simulink model "realtime_PID"  (R2024b)
settings: Solver=ode5  StartTime=0.0  StopTime=10  FixedStep=0.001  RelTol=1e-3
values from neighbouring files (symbols this model uses):
  Beq = 1.223604206496999e-06    (= 1.2236042065e-06)    [DesignPart567.m]    (also in DesignPart9Sine.m; DesignPart9Step.m; Init.m; Real_time_parameter_estimation.m = (data.Beq_hat_pos + data.Beq_hat_neg)/2)
  k_drv = (1 + drv.R3/drv.R4) * drv.R2/(drv.R1 + drv.R2)    [Init.m]
  Kd = Kp * Td    [Init.m]
  Ki = Kp / Ti    [Init.m]
  Kp = deltak * cos(deltaphi)    [Init.m]
  Kw = 1/Tw    (= 33.3333333333)    [Init.m]
  rpm2rads = 2*pi/60    (= 0.10471975512)    [Init.m]
  Tau_sf = 0.005709536387019    (= 0.00570953638702)    [DesignPart567.m]    (also in DesignPart9Sine.m; DesignPart9Step.m; Init.m; State_space_1324.m)
  tl = 1/(3*wgc)    [Init.m]
undefined symbols (not defined in the file or in its folder): gbox, mot, National_Instruments, PCI, sens
libraries: sldrtlib x7, simulink x1
settings Model: SimulationMode=external  ExtModeTrigDuration=1000001  Creator=galeazzolu  LastModifiedBy=lucag
settings DataIOCC: ReturnWorkspaceOutputs=off
settings HardwareCC: ProdBitPerLong=64  ProdHWDeviceType=Intel->x86-64 (Linux 64)
settings RTWCC: Description=Simulink Desktop Real-Time  SystemTargetFile=sldrt.tlc  TemplateMakefile=sldrt.tmf  RTWCompilerOptimization=on
settings CodeAppCC: MaxIdLength=95
settings SimulinkDesktopRealTimeCC: TargetLibSuffix=_sldrt.a  TargetPreCompLibLocation=C:\Program Files\MATLAB\R2024b\toolbox\sldrt\lib\win64  ParMdlRefBuildCompliant=on

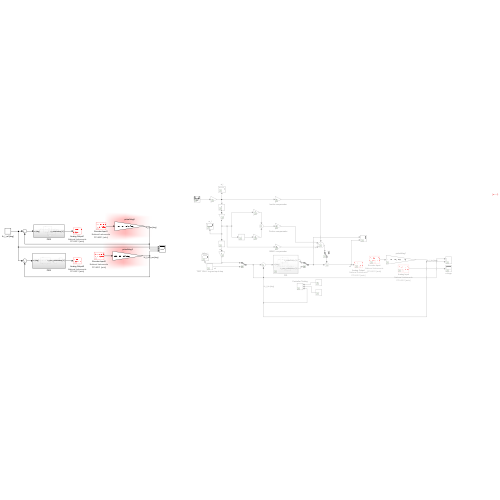
[thumbnail: Simulink's stored preview of the top-level diagram]
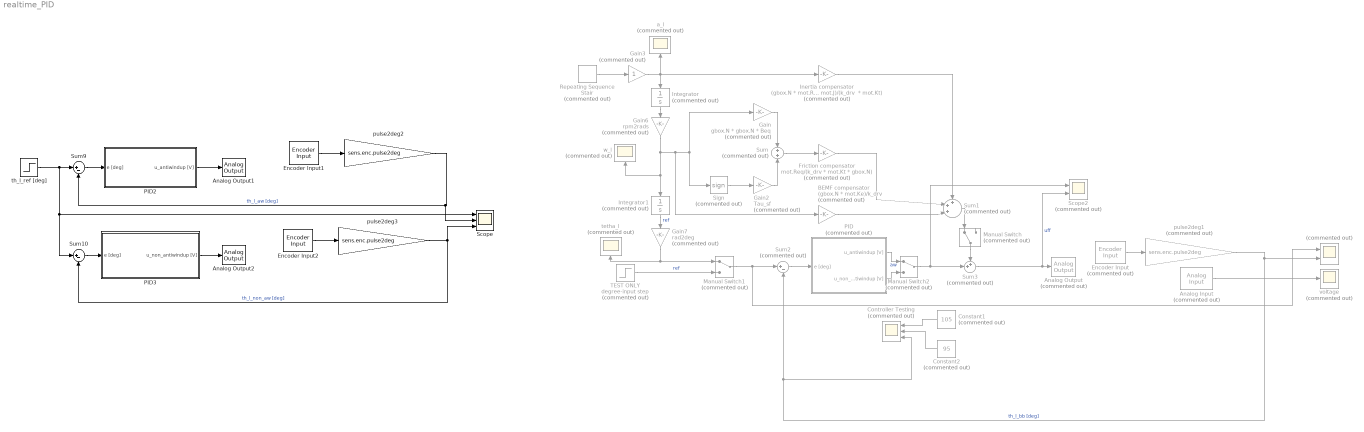
== system realtime_PID ==
  " " : Scope  Commented=on  NumInputPorts=2
  " a_l" : Scope  Commented=on
  " tetha_l" : Scope  Commented=on
  " w_l" : Scope  Commented=on
  Analog Input : sldrtlib/Analog Input  Commented=on  SampleTime=-1  MaxMissedTicks=10  ShowMissedTicks=off  YieldWhenWaiting=off  DrvName=National_Instruments/PCI-6221  DrvAddress=4294967295  DrvOptions=[0 0 0 2 0]  Channels=[1,2]  RangeMode=1  VoltRange=1  DataType=1
      settings: AttributesFormatString=National Instruments\nPCI-6221 [auto]
  Analog Output : sldrtlib/Analog Output  Commented=on  SampleTime=-1  MaxMissedTicks=10  ShowMissedTicks=off  YieldWhenWaiting=off  DrvName=National_Instruments/PCI-6221  DrvAddress=4294967295  DrvOptions=[0 0 0 2 0]  Channels=1  RangeMode=1  VoltRange=1  InitialValue=0  FinalValue=0
      settings: AttributesFormatString=National Instruments\nPCI-6221 [auto]
  Analog Output1 : sldrtlib/Analog Output  SampleTime=-1  MaxMissedTicks=10  ShowMissedTicks=off  YieldWhenWaiting=off  DrvName=National_Instruments/PCI-6221  DrvAddress=4294967295  DrvOptions=[0 0 0 2 0]  Channels=1  RangeMode=1  VoltRange=1  InitialValue=0  FinalValue=0
      settings: AttributesFormatString=National Instruments\nPCI-6221 [auto]
  Analog Output2 : sldrtlib/Analog Output  SampleTime=-1  MaxMissedTicks=10  ShowMissedTicks=off  YieldWhenWaiting=off  DrvName=National_Instruments/PCI-6221  DrvAddress=4294967295  DrvOptions=[0 0 0 2 0]  Channels=1  RangeMode=1  VoltRange=1  InitialValue=0  FinalValue=0
      settings: AttributesFormatString=National Instruments\nPCI-6221 [auto]
  BEMF compensator : Gain  Commented=on  Gain=(gbox.N * mot.Ke)/k_drv
  Constant1 : Constant  Commented=on  Value=105
  Constant2 : Constant  Commented=on  Value=95
  Controller Testing : Scope  Commented=on  NumInputPorts=3
  Encoder Input : sldrtlib/Encoder Input  Commented=on  SampleTime=-1  MaxMissedTicks=10  ShowMissedTicks=off  YieldWhenWaiting=off  DrvName=National_Instruments/PCI-6221  DrvAddress=4294967295  DrvOptions=[0 0 0 2 0]  Channels=1  QuadMode=3  IndexPulse=1  InputFilter=Inf  DataType=1
      settings: AttributesFormatString=National Instruments\nPCI-6221 [auto]
  Encoder Input1 : sldrtlib/Encoder Input  SampleTime=-1  MaxMissedTicks=10  ShowMissedTicks=off  YieldWhenWaiting=off  DrvName=National_Instruments/PCI-6221  DrvAddress=4294967295  DrvOptions=[0 0 0 2 0]  Channels=1  QuadMode=3  IndexPulse=1  InputFilter=Inf  DataType=1
      settings: AttributesFormatString=National Instruments\nPCI-6221 [auto]
  Encoder Input2 : sldrtlib/Encoder Input  SampleTime=-1  MaxMissedTicks=10  ShowMissedTicks=off  YieldWhenWaiting=off  DrvName=National_Instruments/PCI-6221  DrvAddress=4294967295  DrvOptions=[0 0 0 2 0]  Channels=1  QuadMode=3  IndexPulse=1  InputFilter=Inf  DataType=1
      settings: AttributesFormatString=National Instruments\nPCI-6221 [auto]
  Friction compensator : Gain  Commented=on  Gain=mot.Req/(k_drv * mot.Kt * gbox.N)
  Gain : Gain  Commented=on  Gain=gbox.N * gbox.N * Beq
  Gain2 : Gain  Commented=on  Gain=Tau_sf
  Gain3 : Gain  Commented=on
  Gain6 : Gain  Commented=on  Gain=rpm2rads
  Gain7 : Gain  Commented=on  Gain=rad2deg
  Inertia compensator : Gain  Commented=on  Gain="(gbox.N * mot.Req * mot.J)/(k_drv  * mot.Kt)"
  Integrator : Integrator  Commented=on
  Integrator1 : Integrator  Commented=on
  Manual Switch : ManualSwitch  Commented=on
  Manual Switch1 : ManualSwitch  Commented=on
  Manual Switch2 : ManualSwitch  Commented=on
  PID : Subsystem  Commented=on
  PID2 : Subsystem
  PID3 : Subsystem
  Repeating Sequence Stair : simulink/Sources/Repeating Sequence Stair  Commented=on  OutValues=[900 0 -900 -900 0 900]  tsamp=0.5  OutMin=[]  OutMax=[]  OutDataTypeStr=double  OutputDataTypeScalingMode=double  OutDataType=fixdt(0,8)  ConRadixGroup=Best Precision: Vector-wise  OutScaling=2^-12
  Scope : Scope  NumInputPorts=3
  Scope2 : Scope  Commented=on  NumInputPorts=2
  Sign : Signum  Commented=on
  Sum : Sum  Commented=on  Inputs=+|+
  Sum1 : Sum  Commented=on  Inputs=+++|
  Sum10 : Sum  Inputs=|+-
  Sum2 : Sum  Commented=on  Inputs=|+-
  Sum3 : Sum  Commented=on  Inputs=++|
  Sum9 : Sum  Inputs=|+-
  TEST ONLY degree-input step : Step  Commented=on  After=360  SampleTime=0
  pulse2deg1 : Gain  Commented=on  Gain=sens.enc.pulse2deg
  pulse2deg2 : Gain  Gain=sens.enc.pulse2deg
  pulse2deg3 : Gain  Gain=sens.enc.pulse2deg
  th_l_ref [deg] : Step  After=360  SampleTime=0
  voltage : Scope  Commented=on
  wires:
  Sum/1 -> Friction compensator/1
  Gain7/1 -> " tetha_l"/1, Manual Switch1/1
  Sum3/1 -> Analog Output/1, Scope2/2  "uff"
  Sign/1 -> Gain2/1
  Gain3/1 -> Inertia compensator/1, " a_l"/1, Integrator/1
  Encoder Input/1 -> pulse2deg1/1
  Inertia compensator/1 -> Sum1/1
  Gain/1 -> Sum/1
  Repeating Sequence Stair/1 -> Gain3/1
  Constant1/1 -> Controller Testing/1
  pulse2deg1/1 -> Sum2/2, Controller Testing/3, " "/2  "th_l_bb [deg]"
  Gain6/1 -> BEMF compensator/1, Sign/1, Gain/1, Integrator1/1, " w_l"/1
  Sum2/1 -> PID/1(e [deg])
  Gain2/1 -> Sum/2
  Integrator/1 -> Gain6/1
  BEMF compensator/1 -> Sum1/3
  Constant2/1 -> Controller Testing/2
  Integrator1/1 -> Gain7/1  "ref"
  ? -> ?
  Analog Input/1 -> voltage/1
  Manual Switch/1 -> Sum3/1
  Sum1/1 -> Manual Switch/1
  Friction compensator/1 -> Sum1/2
  TEST ONLY degree-input step/1 -> Manual Switch1/2  "ref"
  Manual Switch1/1 -> " "/1, Sum2/1
  PID/2(u_non_antiwindup [V]) -> Manual Switch2/2
  PID/1(u_antiwindup [V]) -> Manual Switch2/1  "aw"
  Manual Switch2/1 -> Scope2/1, Sum3/2
  Sum10/1 -> PID3/1(e [deg])
  Encoder Input2/1 -> pulse2deg3/1
  pulse2deg2/1 -> Scope/2, Sum9/2  "th_l_aw [deg]"
  PID3/1(u_non_antiwindup [V]) -> Analog Output2/1
  Sum9/1 -> PID2/1(e [deg])
  PID2/1(u_antiwindup [V]) -> Analog Output1/1
  pulse2deg3/1 -> Scope/3, Sum10/2  "th_l_non_aw [deg]"
  Encoder Input1/1 -> pulse2deg2/1
  th_l_ref [deg]/1 -> Scope/1, Sum10/1, Sum9/1

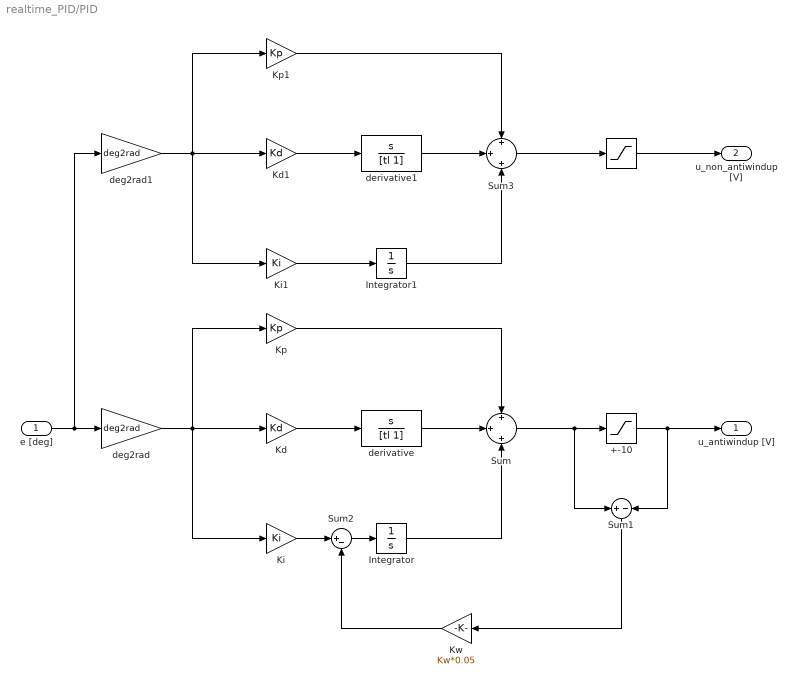
== system realtime_PID/PID ==
  e [deg] : Inport
  " " : Saturate  UpperLimit=10  LowerLimit=-10
  +-10 : Saturate  UpperLimit=10  LowerLimit=-10
  Integrator : Integrator
  Integrator1 : Integrator
  Kd : Gain  Gain=Kd
  Kd1 : Gain  Gain=Kd
  Ki : Gain  Gain=Ki
  Ki1 : Gain  Gain=Ki
  Kp : Gain  Gain=Kp
  Kp1 : Gain  Gain=Kp
  Kw : Gain  Gain=Kw*0.05
  Sum : Sum  Inputs=+|+|+
  Sum1 : Sum  Inputs=+|-
  Sum2 : Sum  Inputs=|+-
  Sum3 : Sum  Inputs=+|+|+
  deg2rad : Gain  Gain=deg2rad
  deg2rad1 : Gain  Gain=deg2rad
  derivative : TransferFcn  Numerator=[1 0]  Denominator=[tl 1]
  derivative1 : TransferFcn  Numerator=[1 0]  Denominator=[tl 1]
  u_antiwindup [V] : Outport
  u_non_antiwindup [V] : Outport  Port=2
  wires:
  e [deg]/1 -> deg2rad1/1, deg2rad/1
  deg2rad/1 -> Kp/1, Ki/1, Kd/1
  Ki/1 -> Sum2/1
  Kp/1 -> Sum/1
  Integrator/1 -> Sum/3
  Kd/1 -> derivative/1
  derivative/1 -> Sum/2
  Sum/1 -> Sum1/1, +-10/1
  Sum2/1 -> Integrator/1
  Sum1/1 -> Kw/1
  Kw/1 -> Sum2/2
  +-10/1 -> u_antiwindup [V]/1, Sum1/2
  deg2rad1/1 -> Kp1/1, Ki1/1, Kd1/1
  Sum3/1 -> " "/1
  derivative1/1 -> Sum3/2
  Kd1/1 -> derivative1/1
  Ki1/1 -> Integrator1/1
  Kp1/1 -> Sum3/1
  Integrator1/1 -> Sum3/3
  " "/1 -> u_non_antiwindup [V]/1

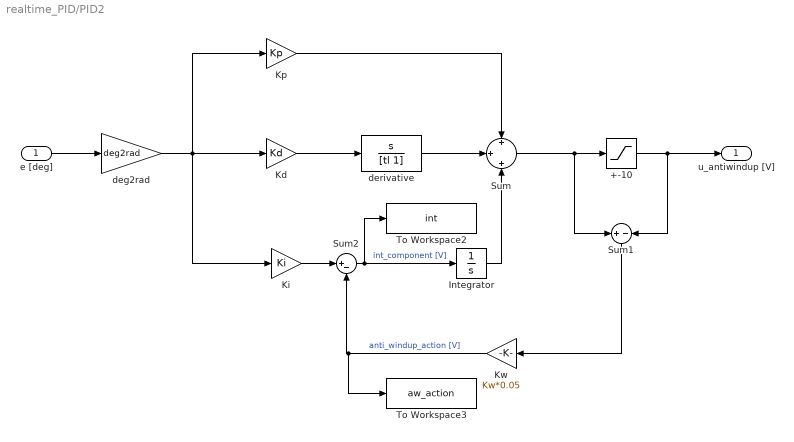
== system realtime_PID/PID2 ==
  e [deg] : Inport
  +-10 : Saturate  UpperLimit=10  LowerLimit=-10
  Integrator : Integrator
  Kd : Gain  Gain=Kd
  Ki : Gain  Gain=Ki
  Kp : Gain  Gain=Kp
  Kw : Gain  Gain=Kw*0.05
  Sum : Sum  Inputs=+|+|+
  Sum1 : Sum  Inputs=+|-
  Sum2 : Sum  Inputs=|+-
  To Workspace2 : ToWorkspace  VariableName=int  SaveFormat=Structure With Time  SampleTime=-1
  To Workspace3 : ToWorkspace  VariableName=aw_action  SaveFormat=Structure With Time  SampleTime=-1
  deg2rad : Gain  Gain=deg2rad
  derivative : TransferFcn  Numerator=[1 0]  Denominator=[tl 1]
  u_antiwindup [V] : Outport
  wires:
  +-10/1 -> Sum1/2, u_antiwindup [V]/1
  Kw/1 -> To Workspace3/1, Sum2/2  "anti_windup_action [V]"
  Sum1/1 -> Kw/1
  Sum2/1 -> To Workspace2/1, Integrator/1  "int_component [V]"
  Sum/1 -> +-10/1, Sum1/1
  derivative/1 -> Sum/2
  Kd/1 -> derivative/1
  Integrator/1 -> Sum/3
  Kp/1 -> Sum/1
  Ki/1 -> Sum2/1
  deg2rad/1 -> Kd/1, Ki/1, Kp/1
  e [deg]/1 -> deg2rad/1

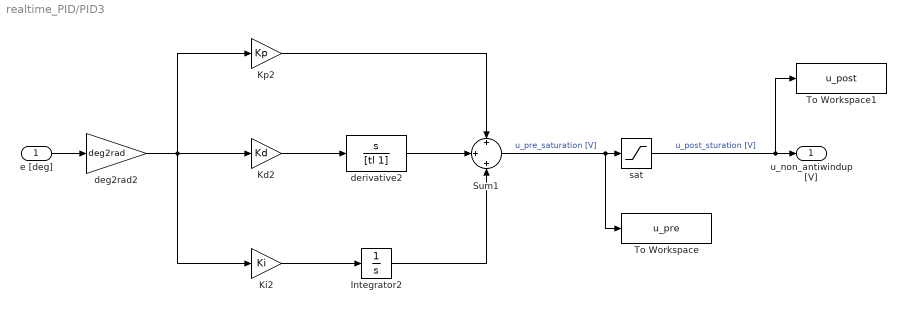
== system realtime_PID/PID3 ==
  e [deg] : Inport
  " sat" : Saturate  UpperLimit=10  LowerLimit=-10
  Integrator2 : Integrator
  Kd2 : Gain  Gain=Kd
  Ki2 : Gain  Gain=Ki
  Kp2 : Gain  Gain=Kp
  Sum1 : Sum  Inputs=+|+|+
  To Workspace : ToWorkspace  VariableName=u_pre  SaveFormat=Structure With Time  SampleTime=-1
  To Workspace1 : ToWorkspace  VariableName=u_post  SaveFormat=Structure With Time  SampleTime=-1
  deg2rad2 : Gain  Gain=deg2rad
  derivative2 : TransferFcn  Numerator=[1 0]  Denominator=[tl 1]
  u_non_antiwindup [V] : Outport
  wires:
  Integrator2/1 -> Sum1/3
  Kd2/1 -> derivative2/1
  deg2rad2/1 -> Kd2/1, Ki2/1, Kp2/1
  Kp2/1 -> Sum1/1
  derivative2/1 -> Sum1/2
  " sat"/1 -> To Workspace1/1, u_non_antiwindup [V]/1  "u_post_sturation [V]"
  Ki2/1 -> Integrator2/1
  Sum1/1 -> To Workspace/1, " sat"/1  "u_pre_saturation [V]"
  e [deg]/1 -> deg2rad2/1
